simulink model "stage_two"  (R2021b)
settings: Solver=VariableStepAuto  StartTime=0.0  StopTime=0.2  FixedStep=1e3  RelTol=1e-8
libraries: spsTriangleGeneratorLib x1
settings Model: Creator=Selected  LastModifiedBy=Selected
settings SolverCC: ShapePreserveControl=EnableAll

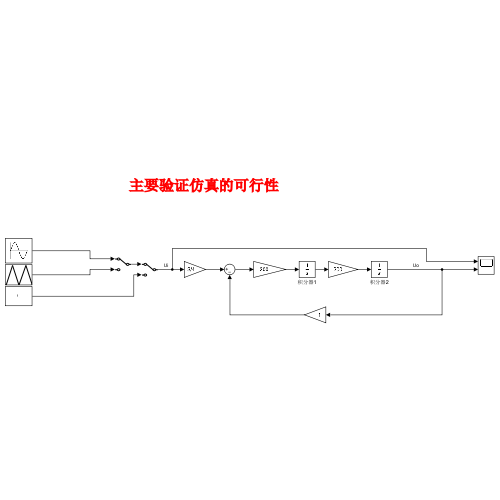
[thumbnail: Simulink's stored preview of the top-level diagram]
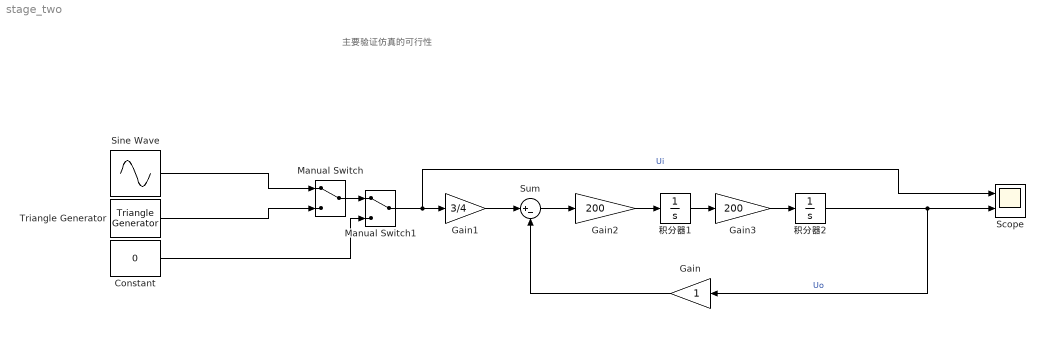
== system stage_two ==
  note: 主要验证仿真的可行性
  Constant : Constant  Value=0
  Gain : Gain
  Gain1 : Gain  Gain=3/4
  Gain2 : Gain  Gain=200
  Gain3 : Gain  Gain=200
  Manual Switch : ManualSwitch
  Manual Switch1 : ManualSwitch
  Scope : Scope  NumInputPorts=2
  Sine Wave : Sin  Amplitude=2  Frequency=600  SampleTime=0
  Sum : Sum  Inputs=|+-
  Triangle Generator : spsTriangleGeneratorLib/Triangle Generator  Freq=600/2/pi  Phase=0  Ts=0
  积分器1 : Integrator
  积分器2 : Integrator  InitialCondition=1
  wires:
  积分器2/1 -> Gain/1, Scope/2  "Uo"
  Gain/1 -> Sum/2
  Gain1/1 -> Sum/1
  Manual Switch/1 -> Manual Switch1/1
  Sine Wave/1 -> Manual Switch/1
  Manual Switch1/1 -> Scope/1, Gain1/1  "Ui"
  Constant/1 -> Manual Switch1/2
  Triangle Generator/1 -> Manual Switch/2
  Sum/1 -> Gain2/1
  Gain2/1 -> 积分器1/1
  积分器1/1 -> Gain3/1
  Gain3/1 -> 积分器2/1
